simulink library "Fricciones"  (Simulink 8.3)
settings: Solver=ode45  StartTime=0.0  StopTime=10.0  RelTol=1e-3
values from neighbouring files (symbols this model uses):
  Fc = 0.005    [matlab.mat]
  Fs = 0.01    [matlab.mat]
undefined symbols (not defined in the file or in its folder): Friccion, mu_pts, Normal_Force_Pist_Cyl
undefined symbols (not defined in the file): Fsc, MUK, MUS, VTH
libraries: nesl_utility x17, fl_lib x14, Fricciones x4, MS2G_SS_Intf_Lib x4
settings Model: Creator=Sebastian  LastModifiedBy=Sebastian

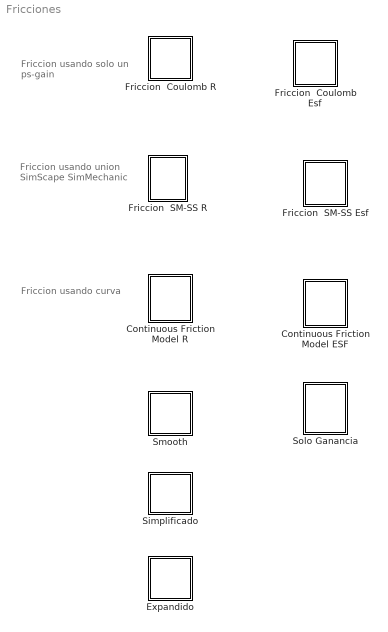
== system Fricciones ==
  note: Friccion
      |  usando curva
  note: Friccion usando
      | union SimScape
      | SimMechanic
  note: Friccion usando
      | solo un ps-gain
  Continuous Friction Model ESF : Subsystem  mask{muk=MUK, mus=MUS, vth=VTH}
      mask prompts: muk "Coefficient of kinetic friction"; mus "Coefficient of static friction"; vth "Velocity threshold"
      mask help: Continuous friction model interpolates between low-speed quasi-static friction and higher-speed kinetic friction.
      mask init:
      | %%FRICTION CURVE
      | % Velocity vs. coefficient of friction
      | 
      | % NUMBER OF POINTS ON CURVE
      | num_fs_pts = 101;
      | 
      | % CURVE LIMITS
      | v_lowlim = -3*vth;
      | v_upplim = 3*vth;
      | 
      | % GENERATE X-AXIS POINTS (velocity)
      | v_pts = linspace(v_lowlim, v_upplim, num_fs_pts);
      | 
      | % DETERMINE Y-AXIS POINTS (coefficient of friction)
      | for i=1:num_fs_pts
      |     if(v_pts(i)<(-1.5*vth))
      |         mu_pts(i) = -muk;
      |     elseif(v_pts(i)>=-1.5*vth && v_pts(i)<-vth)
      |         mu_pts(i) = -(muk-mus)/(0.5*vth)*(-1.5*vth-v_pts(i))-muk;
      |     elseif(v_pts(i)>=-vth && v_pts(i)<vth)
      |         mu_pts(i) = -(mus)/vth*(-vth-v_pts(i))-mus;
      |     elseif(v_pts(i)>=vth && v_pts(i)<1.5*vth)
      |         mu_pts(i) = (muk-mus)/(0.5*vth)*(v_pts(i)-1.5*vth)+muk;
      |     elseif(v_pts(i)>=(1.5*vth))
      |         mu_pts(i) = muk;
      |     end
      | end
  Continuous Friction Model R : Subsystem  mask{muk=Fc, mus=Fs, vth=0}
      mask init:
      | %%FRICTION CURVE
      | % Velocity vs. coefficient of friction
      | 
      | % NUMBER OF POINTS ON CURVE
      | num_fs_pts = 101;
      | 
      | % CURVE LIMITS
      | v_lowlim = -3*vth;
      | v_upplim = 3*vth;
      | 
      | % GENERATE X-AXIS POINTS (velocity)
      | v_pts = linspace(v_lowlim, v_upplim, num_fs_pts);
      | 
      | % DETERMINE Y-AXIS POINTS (coefficient of friction)
      | for i=1:num_fs_pts
      |     if(v_pts(i)<(-1.5*vth))
      |         mu_pts(i) = -muk;
      |     elseif(v_pts(i)>=-1.5*vth && v_pts(i)<-vth)
      |         mu_pts(i) = -(muk-mus)/(0.5*vth)*(-1.5*vth-v_pts(i))-muk;
      |     elseif(v_pts(i)>=-vth && v_pts(i)<vth)
      |         mu_pts(i) = -(mus)/vth*(-vth-v_pts(i))-mus;
      |     elseif(v_pts(i)>=vth && v_pts(i)<1.5*vth)
      |         mu_pts(i) = (muk-mus)/(0.5*vth)*(v_pts(i)-1.5*vth)+muk;
      |     elseif(v_pts(i)>=(1.5*vth))
      |         mu_pts(i) = muk;
      |     end
      | end
  Expandido : Subsystem
      mask init:
      | To=0.1
      | Fm=0.2
  Friccion  Coulomb Esf : Subsystem
  Friccion  Coulomb R : Subsystem
  Friccion  SM-SS Esf : Subsystem  mask{BFT=0.2, CFT=0.15, VFc=0.001, Tac=5}
      mask prompts: BFT "Breakaway friction torque (N*m)"; CFT "Coulomb friction torque (N*m)"; VFc "Viscous friction coeff (N*m/(rad/s))"; Tac "Transition approximation coeff (s/rad)"
  Friccion  SM-SS R : Subsystem  mask{BFT=Fs, CFT=Fc, VFc=Fsc, Tac=5}
      mask prompts: BFT "Breakaway friction torque (N*m)"; CFT "Coulomb friction torque (N*m)"; VFc "Viscous friction coeff (N*m/(rad/s))"; Tac "Transition approximation coeff (s/rad)"
  Simplificado : Subsystem
  Smooth : Subsystem
      mask init:
      | C1=15;
      | C2=1.5;
      | C3=900;
  Solo Ganancia : Subsystem

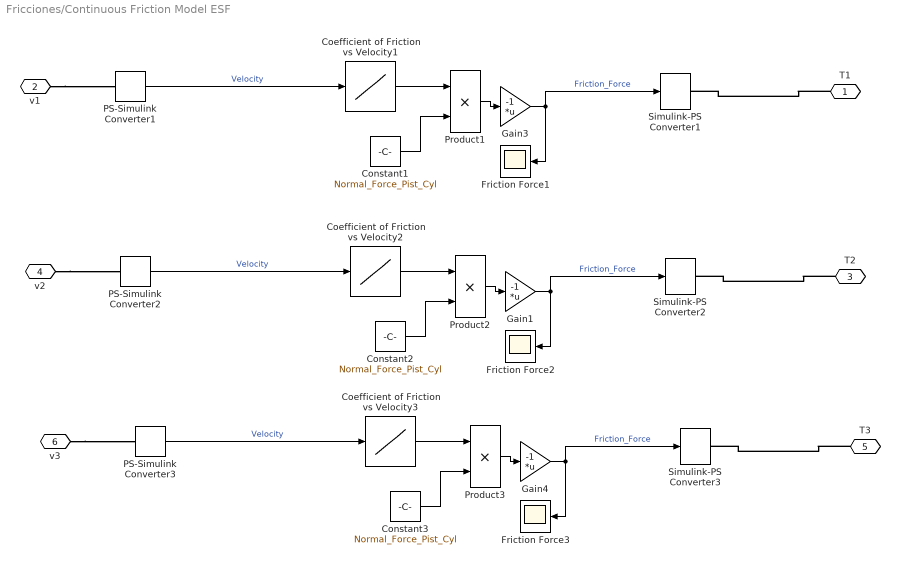
== system Fricciones/Continuous Friction Model ESF ==
  Coefficient of Friction vs Velocity1 : Lookup  InputValues=v_pts  Table=mu_pts
  Coefficient of Friction vs Velocity2 : Lookup  InputValues=v_pts  Table=mu_pts
  Coefficient of Friction vs Velocity3 : Lookup  InputValues=v_pts  Table=mu_pts
  Constant1 : Constant  Value=Normal_Force_Pist_Cyl
  Constant2 : Constant  Value=Normal_Force_Pist_Cyl
  Constant3 : Constant  Value=Normal_Force_Pist_Cyl
  Friction Force1 : Scope
      settings: TimeRange=10  YMin=-10  YMax=10  SaveName=ScopeData8
  Friction Force2 : Scope
      settings: TimeRange=10  YMin=-10  YMax=10  SaveName=ScopeData9
  Friction Force3 : Scope
      settings: TimeRange=10  YMin=-10  YMax=10  SaveName=ScopeData10
  Gain1 : Gain  Gain=-1  Multiplication=Matrix(K*u)  SaturateOnIntegerOverflow=on  OutDataTypeStr=Inherit: Same as input  ParamDataTypeStr=Inherit: Same as input
  Gain3 : Gain  Gain=-1  Multiplication=Matrix(K*u)  SaturateOnIntegerOverflow=on  OutDataTypeStr=Inherit: Same as input  ParamDataTypeStr=Inherit: Same as input
  Gain4 : Gain  Gain=-1  Multiplication=Matrix(K*u)  SaturateOnIntegerOverflow=on  OutDataTypeStr=Inherit: Same as input  ParamDataTypeStr=Inherit: Same as input
  PS-Simulink Converter1 : nesl_utility/PS-Simulink Converter  PhysicalDomain=network_engine_domain  SubClassName=ps_output  LeftPortType=input  RightPortType=output  PseudoPeriodic=off  Frequencies=[]  Unit=1  AffineConversion=off
  PS-Simulink Converter2 : nesl_utility/PS-Simulink Converter  PhysicalDomain=network_engine_domain  SubClassName=ps_output  LeftPortType=input  RightPortType=output  PseudoPeriodic=off  Frequencies=[]  Unit=1  AffineConversion=off
  PS-Simulink Converter3 : nesl_utility/PS-Simulink Converter  PhysicalDomain=network_engine_domain  SubClassName=ps_output  LeftPortType=input  RightPortType=output  PseudoPeriodic=off  Frequencies=[]  Unit=1  AffineConversion=off
  Product1 : Product  RndMeth=Zero
  Product2 : Product  RndMeth=Zero
  Product3 : Product  RndMeth=Zero
  Simulink-PS Converter1 : nesl_utility/Simulink-PS Converter  PhysicalDomain=network_engine_domain  SubClassName=ps_input  LeftPortType=input  RightPortType=output  PseudoPeriodic=off  Frequencies=[]  NoiseDistribution=none  NoiseParameters=[]  Unit=1  AffineConversion=off  InputFiltering=off  SimscapeFilterOrder=1  InputFilterTimeConstant=0.001  UdotUserProvided=1
  Simulink-PS Converter2 : nesl_utility/Simulink-PS Converter  PhysicalDomain=network_engine_domain  SubClassName=ps_input  LeftPortType=input  RightPortType=output  PseudoPeriodic=off  Frequencies=[]  NoiseDistribution=none  NoiseParameters=[]  Unit=1  AffineConversion=off  InputFiltering=off  SimscapeFilterOrder=1  InputFilterTimeConstant=0.001  UdotUserProvided=1
  Simulink-PS Converter3 : nesl_utility/Simulink-PS Converter  PhysicalDomain=network_engine_domain  SubClassName=ps_input  LeftPortType=input  RightPortType=output  PseudoPeriodic=off  Frequencies=[]  NoiseDistribution=none  NoiseParameters=[]  Unit=1  AffineConversion=off  InputFiltering=off  SimscapeFilterOrder=1  InputFilterTimeConstant=0.001  UdotUserProvided=1
  T1 : PMIOPort  Port=1  Side=Left
  v1 : PMIOPort  Port=2  Side=Right
  T2 : PMIOPort  Port=3  Side=Left
  v2 : PMIOPort  Port=4  Side=Right
  T3 : PMIOPort  Port=5  Side=Left
  v3 : PMIOPort  Port=6  Side=Right
  wires:
  Constant1/1 -> Product1/2
  Coefficient of Friction vs Velocity1/1 -> Product1/1
  PS-Simulink Converter1/1 -> Coefficient of Friction vs Velocity1/1  "Velocity"
  Product1/1 -> Gain3/1
  Gain3/1 -> Simulink-PS Converter1/1, Friction Force1/1  "Friction_Force"
  Constant2/1 -> Product2/2
  Coefficient of Friction vs Velocity2/1 -> Product2/1
  PS-Simulink Converter2/1 -> Coefficient of Friction vs Velocity2/1  "Velocity"
  Product2/1 -> Gain1/1
  Gain1/1 -> Simulink-PS Converter2/1, Friction Force2/1  "Friction_Force"
  Constant3/1 -> Product3/2
  Coefficient of Friction vs Velocity3/1 -> Product3/1
  PS-Simulink Converter3/1 -> Coefficient of Friction vs Velocity3/1  "Velocity"
  Product3/1 -> Gain4/1
  Gain4/1 -> Simulink-PS Converter3/1, Friction Force3/1  "Friction_Force"
  connections:
  T2/RConn1 -- Simulink-PS Converter2/RConn1
  v2/RConn1 -- PS-Simulink Converter2/LConn1
  v1/RConn1 -- PS-Simulink Converter1/LConn1
  T1/RConn1 -- Simulink-PS Converter1/RConn1
  v3/RConn1 -- PS-Simulink Converter3/LConn1
  T3/RConn1 -- Simulink-PS Converter3/RConn1

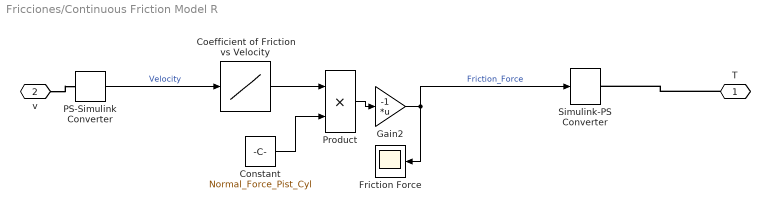
== system Fricciones/Continuous Friction Model R ==
  Coefficient of Friction vs Velocity : Lookup  InputValues=v_pts  Table=mu_pts
  Constant : Constant  Value=Normal_Force_Pist_Cyl
  Friction Force : Scope
      settings: TimeRange=10  YMin=-10  YMax=10  SaveName=ScopeData4
  Gain2 : Gain  Gain=-1  Multiplication=Matrix(K*u)  SaturateOnIntegerOverflow=on  OutDataTypeStr=Inherit: Same as input  ParamDataTypeStr=Inherit: Same as input
  PS-Simulink Converter : nesl_utility/PS-Simulink Converter  PhysicalDomain=network_engine_domain  SubClassName=ps_output  LeftPortType=input  RightPortType=output  PseudoPeriodic=off  Frequencies=[]  Unit=1  AffineConversion=off
  Product : Product  RndMeth=Zero
  Simulink-PS Converter : nesl_utility/Simulink-PS Converter  PhysicalDomain=network_engine_domain  SubClassName=ps_input  LeftPortType=input  RightPortType=output  PseudoPeriodic=off  Frequencies=[]  NoiseDistribution=none  NoiseParameters=[]  Unit=1  AffineConversion=off  InputFiltering=off  SimscapeFilterOrder=1  InputFilterTimeConstant=0.001  UdotUserProvided=1
  T : PMIOPort  Port=1  Side=Right
  v : PMIOPort  Port=2  Side=Right
  wires:
  PS-Simulink Converter/1 -> Coefficient of Friction vs Velocity/1  "Velocity"
  Coefficient of Friction vs Velocity/1 -> Product/1
  Product/1 -> Gain2/1
  Gain2/1 -> Simulink-PS Converter/1, Friction Force/1  "Friction_Force"
  Constant/1 -> Product/2
  connections:
  v/RConn1 -- PS-Simulink Converter/LConn1
  T/RConn1 -- Simulink-PS Converter/RConn1

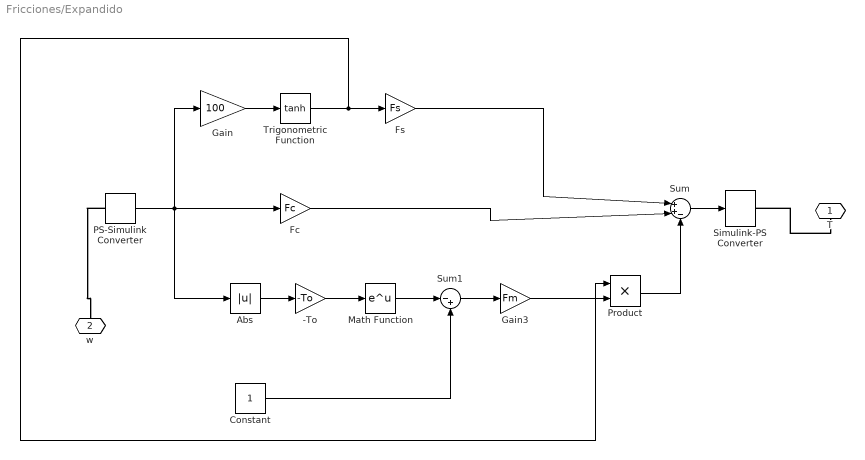
== system Fricciones/Expandido ==
  -To : Gain  Gain=-To
  Abs : Abs
  Constant : Constant
  Fc : Gain  Gain=Fc
  Fs : Gain  Gain=Fs
  Gain : Gain  Gain=100
  Gain3 : Gain  Gain=Fm
  Math Function : Math  SaturateOnIntegerOverflow=on
  PS-Simulink Converter : nesl_utility/PS-Simulink Converter  PhysicalDomain=network_engine_domain  SubClassName=ps_output  LeftPortType=input  RightPortType=output  PseudoPeriodic=off  Frequencies=[]  Unit=1  AffineConversion=off
  Product : Product
  Simulink-PS Converter : nesl_utility/Simulink-PS Converter  PhysicalDomain=network_engine_domain  SubClassName=ps_input  LeftPortType=input  RightPortType=output  PseudoPeriodic=off  Frequencies=[]  NoiseDistribution=none  NoiseParameters=[]  Unit=1  AffineConversion=off  InputFiltering=off  SimscapeFilterOrder=1  InputFilterTimeConstant=0.001  UdotUserProvided=1
  Sum : Sum  Inputs=|++-
  Sum1 : Sum  Inputs=|-+
  Trigonometric Function : Trigonometry  Operator=tanh
  T : PMIOPort  Port=1  Side=Left
  w : PMIOPort  Port=2  Side=Right
  wires:
  Gain/1 -> Trigonometric Function/1
  Trigonometric Function/1 -> Product/1, Fs/1
  PS-Simulink Converter/1 -> Abs/1, Fc/1, Gain/1
  Fs/1 -> Sum/1
  Fc/1 -> Sum/2
  Abs/1 -> -To/1
  -To/1 -> Math Function/1
  Math Function/1 -> Sum1/1
  Constant/1 -> Sum1/2
  Sum1/1 -> Gain3/1
  Gain3/1 -> Product/2
  Product/1 -> Sum/3
  Sum/1 -> Simulink-PS Converter/1
  connections:
  PS-Simulink Converter/LConn1 -- w/RConn1
  T/RConn1 -- Simulink-PS Converter/RConn1

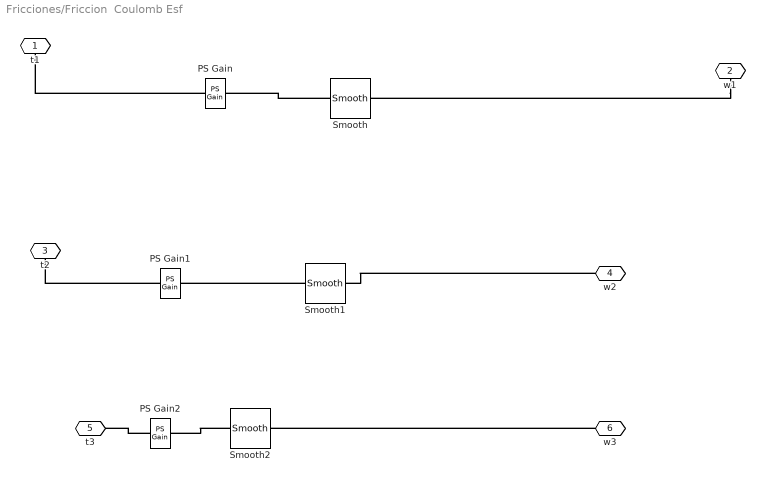
== system Fricciones/Friccion  Coulomb Esf ==
  PS Gain : fl_lib/Physical Signals/Functions/PS Gain  gain=-1
  PS Gain1 : fl_lib/Physical Signals/Functions/PS Gain  gain=-1
  PS Gain2 : fl_lib/Physical Signals/Functions/PS Gain  gain=-1
  Smooth : Fricciones/Smooth  SystemSampleTime=-1
  Smooth1 : Fricciones/Smooth  SystemSampleTime=-1
  Smooth2 : Fricciones/Smooth  SystemSampleTime=-1
  t1 : PMIOPort  Port=1  Side=Left
  w1 : PMIOPort  Port=2  Side=Right
  t2 : PMIOPort  Port=3  Side=Left
  w2 : PMIOPort  Port=4  Side=Right
  t3 : PMIOPort  Port=5  Side=Left
  w3 : PMIOPort  Port=6  Side=Right
  connections:
  w3/RConn1 -- Smooth2/RConn1
  w2/RConn1 -- Smooth1/RConn1
  w1/RConn1 -- Smooth/RConn1
  Smooth2/LConn1 -- PS Gain2/LConn1
  PS Gain2/RConn1 -- t3/RConn1
  Smooth1/LConn1 -- PS Gain1/LConn1
  PS Gain1/RConn1 -- t2/RConn1
  Smooth/LConn1 -- PS Gain/LConn1
  PS Gain/RConn1 -- t1/RConn1

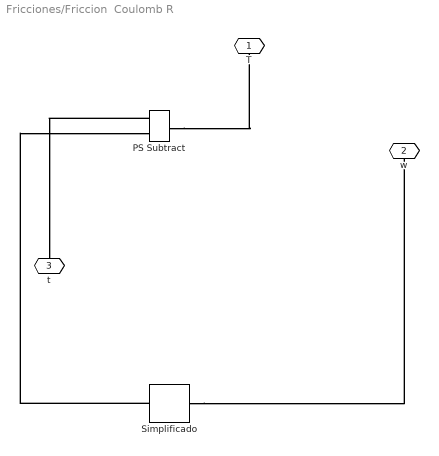
== system Fricciones/Friccion  Coulomb R ==
  PS Subtract : fl_lib/Physical Signals/Functions/PS Subtract
  Simplificado : Fricciones/Simplificado
  T : PMIOPort  Port=1  Side=Right
  w : PMIOPort  Port=2  Side=Right
  t : PMIOPort  Port=3  Side=Left
  connections:
  PS Subtract/LConn1 -- t/RConn1
  PS Subtract/RConn1 -- T/RConn1
  Simplificado/RConn1 -- w/RConn1
  Simplificado/LConn1 -- PS Subtract/LConn2

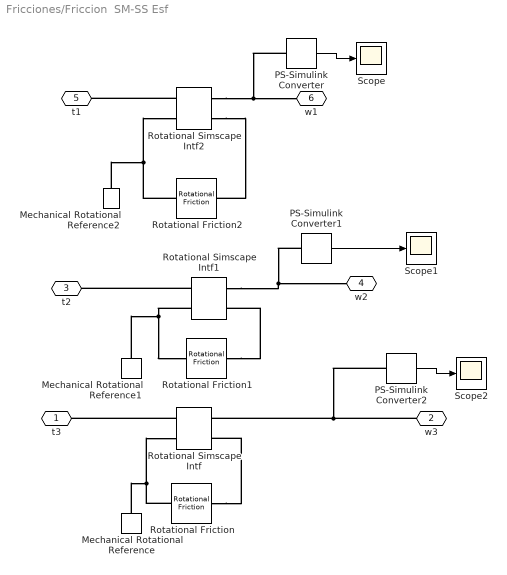
== system Fricciones/Friccion  SM-SS Esf ==
  Mechanical Rotational Reference : fl_lib/Mechanical/Rotational Elements/Mechanical Rotational Reference
  Mechanical Rotational Reference1 : fl_lib/Mechanical/Rotational Elements/Mechanical Rotational Reference
  Mechanical Rotational Reference2 : fl_lib/Mechanical/Rotational Elements/Mechanical Rotational Reference
  PS-Simulink Converter : nesl_utility/PS-Simulink Converter  PhysicalDomain=network_engine_domain  SubClassName=ps_output  LeftPortType=input  RightPortType=output  PseudoPeriodic=off  Frequencies=[]  Unit=rad/s  AffineConversion=off
  PS-Simulink Converter1 : nesl_utility/PS-Simulink Converter  PhysicalDomain=network_engine_domain  SubClassName=ps_output  LeftPortType=input  RightPortType=output  PseudoPeriodic=off  Frequencies=[]  Unit=rad/s  AffineConversion=off
  PS-Simulink Converter2 : nesl_utility/PS-Simulink Converter  PhysicalDomain=network_engine_domain  SubClassName=ps_output  LeftPortType=input  RightPortType=output  PseudoPeriodic=off  Frequencies=[]  Unit=rad/s  AffineConversion=off
  Rotational Simscape Intf : MS2G_SS_Intf_Lib/Rotational Simscape Intf
  Rotational Simscape Intf1 : MS2G_SS_Intf_Lib/Rotational Simscape Intf
  Rotational Simscape Intf2 : MS2G_SS_Intf_Lib/Rotational Simscape Intf
  Rotational Friction : fl_lib/Mechanical/Rotational Elements/Rotational Friction  brkwy_trq=BFT N*m  Col_trq=CFT N*m  visc_coef=VFc N*m/(rad/s)  trans_coef=Tac s/rad  vel_thr=1e-4 rad/s  w_specify=on  w_priority=High  w=0 rad/s  t_specify=on  t_priority=High  t=0 N*m
  Rotational Friction1 : fl_lib/Mechanical/Rotational Elements/Rotational Friction  brkwy_trq=BFT N*m  Col_trq=CFT N*m  visc_coef=VFc N*m/(rad/s)  trans_coef=Tac s/rad  vel_thr=1e-4 rad/s  w_specify=on  w_priority=High  w=0 rad/s  t_specify=on  t_priority=High  t=0 N*m
  Rotational Friction2 : fl_lib/Mechanical/Rotational Elements/Rotational Friction  brkwy_trq=BFT N*m  Col_trq=CFT N*m  visc_coef=VFc N*m/(rad/s)  trans_coef=Tac s/rad  vel_thr=1e-4 rad/s  w_specify=on  w_priority=High  w=0 rad/s  t_specify=on  t_priority=High  t=0 N*m
  Scope : Scope
      settings: YMin=1.26939e-05  YMax=1.26939e-05
  Scope1 : Scope
      settings: YMin=-0.063  YMax=-0.0525
  Scope2 : Scope
      settings: YMin=1.26939e-05  YMax=1.26939e-05  SaveName=ScopeData2
  t3 : PMIOPort  Port=1  Side=Left
  w3 : PMIOPort  Port=2  Side=Right
  t2 : PMIOPort  Port=3  Side=Left
  w2 : PMIOPort  Port=4  Side=Right
  t1 : PMIOPort  Port=5  Side=Left
  w1 : PMIOPort  Port=6  Side=Right
  wires:
  PS-Simulink Converter1/1 -> Scope1/1
  PS-Simulink Converter/1 -> Scope/1
  PS-Simulink Converter2/1 -> Scope2/1
  connections:
  Rotational Friction/RConn1 -- Rotational Simscape Intf/RConn2 -- Mechanical Rotational Reference/LConn1
  Rotational Friction1/LConn1 -- Rotational Simscape Intf1/LConn2
  Rotational Simscape Intf2/LConn1 -- PS-Simulink Converter/LConn1 -- w1/RConn1
  Rotational Simscape Intf1/LConn1 -- PS-Simulink Converter1/LConn1 -- w2/RConn1
  Rotational Friction2/RConn1 -- Rotational Simscape Intf2/RConn2 -- Mechanical Rotational Reference2/LConn1
  Rotational Simscape Intf2/RConn1 -- t1/RConn1
  Rotational Friction/LConn1 -- Rotational Simscape Intf/LConn2
  w3/RConn1 -- PS-Simulink Converter2/LConn1 -- Rotational Simscape Intf/LConn1
  Rotational Simscape Intf1/RConn2 -- Rotational Friction1/RConn1 -- Mechanical Rotational Reference1/LConn1
  Rotational Simscape Intf/RConn1 -- t3/RConn1
  Rotational Simscape Intf2/LConn2 -- Rotational Friction2/LConn1
  Rotational Simscape Intf1/RConn1 -- t2/RConn1

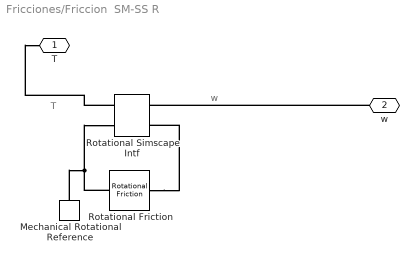
== system Fricciones/Friccion  SM-SS R ==
  note: T
  note: w
  Mechanical Rotational Reference : fl_lib/Mechanical/Rotational Elements/Mechanical Rotational Reference
  Rotational Simscape Intf : MS2G_SS_Intf_Lib/Rotational Simscape Intf
  Rotational Friction : fl_lib/Mechanical/Rotational Elements/Rotational Friction  brkwy_trq=BFT N*m  Col_trq=CFT N*m  visc_coef=VFc N*m/(rad/s)  trans_coef=Tac s/rad  vel_thr=1e-4 rad/s  w_specify=on  w_priority=High  w=0 rad/s  t_specify=on  t_priority=High  t=0 N*m
  T : PMIOPort  Port=1  Side=Right
  w : PMIOPort  Port=2  Side=Right
  connections:
  Rotational Friction/RConn1 -- Rotational Simscape Intf/RConn2 -- Mechanical Rotational Reference/LConn1
  w/RConn1 -- Rotational Simscape Intf/LConn1
  Rotational Friction/LConn1 -- Rotational Simscape Intf/LConn2
  Rotational Simscape Intf/RConn1 -- T/RConn1

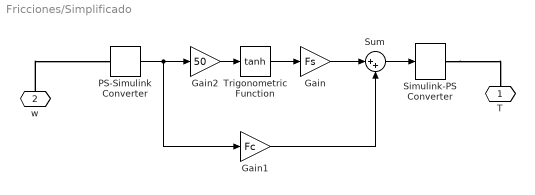
== system Fricciones/Simplificado ==
  Gain : Gain  Gain=Fs
  Gain1 : Gain  Gain=Fc
  Gain2 : Gain  Gain=50
  PS-Simulink Converter : nesl_utility/PS-Simulink Converter  PhysicalDomain=network_engine_domain  SubClassName=ps_output  LeftPortType=input  RightPortType=output  PseudoPeriodic=off  Frequencies=[]  Unit=1  AffineConversion=off
  Simulink-PS Converter : nesl_utility/Simulink-PS Converter  PhysicalDomain=network_engine_domain  SubClassName=ps_input  LeftPortType=input  RightPortType=output  PseudoPeriodic=off  Frequencies=[]  NoiseDistribution=none  NoiseParameters=[]  Unit=1  AffineConversion=off  InputFiltering=off  SimscapeFilterOrder=1  InputFilterTimeConstant=0.001  UdotUserProvided=1
  Sum : Sum  Inputs=|++
  Trigonometric Function : Trigonometry  Operator=tanh
  T : PMIOPort  Port=1  Side=Left
  w : PMIOPort  Port=2  Side=Right
  wires:
  Sum/1 -> Simulink-PS Converter/1
  PS-Simulink Converter/1 -> Gain2/1, Gain1/1
  Gain/1 -> Sum/1
  Gain1/1 -> Sum/2
  Gain2/1 -> Trigonometric Function/1
  Trigonometric Function/1 -> Gain/1
  connections:
  w/RConn1 -- PS-Simulink Converter/LConn1
  Simulink-PS Converter/RConn1 -- T/RConn1

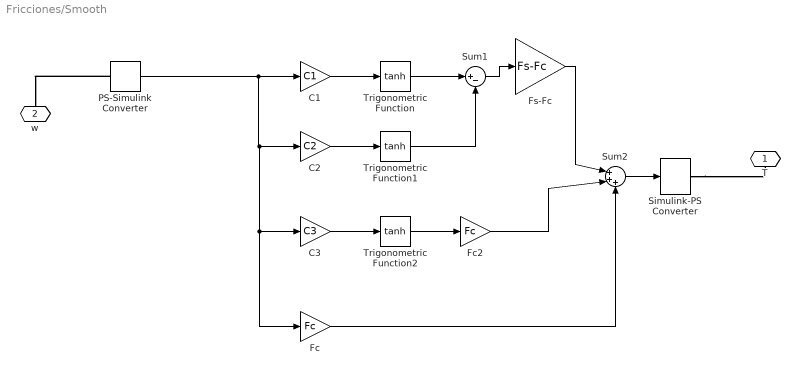
== system Fricciones/Smooth ==
  C1 : Gain  Gain=C1
  C2 : Gain  Gain=C2
  C3 : Gain  Gain=C3
  Fc : Gain  Gain=Fc
  Fc2 : Gain  Gain=Fc
  Fs-Fc : Gain  Gain=Fs-Fc
  PS-Simulink Converter : nesl_utility/PS-Simulink Converter  PhysicalDomain=network_engine_domain  SubClassName=ps_output  LeftPortType=input  RightPortType=output  PseudoPeriodic=off  Frequencies=[]  Unit=1  AffineConversion=off
  Simulink-PS Converter : nesl_utility/Simulink-PS Converter  PhysicalDomain=network_engine_domain  SubClassName=ps_input  LeftPortType=input  RightPortType=output  PseudoPeriodic=off  Frequencies=[]  NoiseDistribution=none  NoiseParameters=[]  Unit=1  AffineConversion=off  InputFiltering=off  SimscapeFilterOrder=1  InputFilterTimeConstant=0.001  UdotUserProvided=1
  Sum1 : Sum  Inputs=|+-
  Sum2 : Sum  Inputs=|+++
  Trigonometric Function : Trigonometry  Operator=tanh
  Trigonometric Function1 : Trigonometry  Operator=tanh
  Trigonometric Function2 : Trigonometry  Operator=tanh
  T : PMIOPort  Port=1  Side=Left
  w : PMIOPort  Port=2  Side=Right
  wires:
  PS-Simulink Converter/1 -> Fc/1, C3/1, C2/1, C1/1
  Trigonometric Function/1 -> Sum1/1
  Trigonometric Function2/1 -> Fc2/1
  Sum1/1 -> Fs-Fc/1
  Trigonometric Function1/1 -> Sum1/2
  C3/1 -> Trigonometric Function2/1
  Fs-Fc/1 -> Sum2/1
  Fc2/1 -> Sum2/2
  Fc/1 -> Sum2/3
  C2/1 -> Trigonometric Function1/1
  C1/1 -> Trigonometric Function/1
  Sum2/1 -> Simulink-PS Converter/1
  connections:
  PS-Simulink Converter/LConn1 -- w/RConn1
  Simulink-PS Converter/RConn1 -- T/RConn1

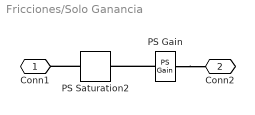
== system Fricciones/Solo Ganancia ==
  PS Gain : fl_lib/Physical Signals/Functions/PS Gain  gain=-Friccion
  PS Saturation2 : fl_lib/Physical Signals/Nonlinear Operators/PS Saturation  upper_limit=0.1  lower_limit=- 0.1
  Conn1 : PMIOPort  Port=1  Side=Left
  Conn2 : PMIOPort  Port=2  Side=Right
  connections:
  PS Gain/RConn1 -- PS Saturation2/LConn1
  PS Saturation2/RConn1 -- Conn1/RConn1
  PS Gain/LConn1 -- Conn2/RConn1
